simulink model "MTTE_TractionControl"  (R2015a)
settings: Solver=ode45  StartTime=0.0  StopTime=10.0  RelTol=1e-3
libraries: simulink x6
settings Model: Creator=Alexander  LastModifiedBy=Alexander

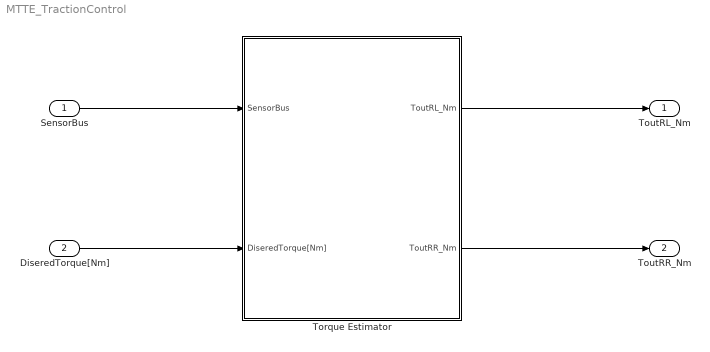
== system MTTE_TractionControl ==
  SensorBus : Inport
  DiseredTorque[Nm] : Inport  Port=2
  Torque Estimator : Subsystem
  ToutRL_Nm : Outport
  ToutRR_Nm : Outport  Port=2
  wires:
  SensorBus/1 -> Torque Estimator/1(SensorBus)
  DiseredTorque[Nm]/1 -> Torque Estimator/2(DiseredTorque[Nm])
  Torque Estimator/1(ToutRL_Nm) -> ToutRL_Nm/1
  Torque Estimator/2(ToutRR_Nm) -> ToutRR_Nm/1

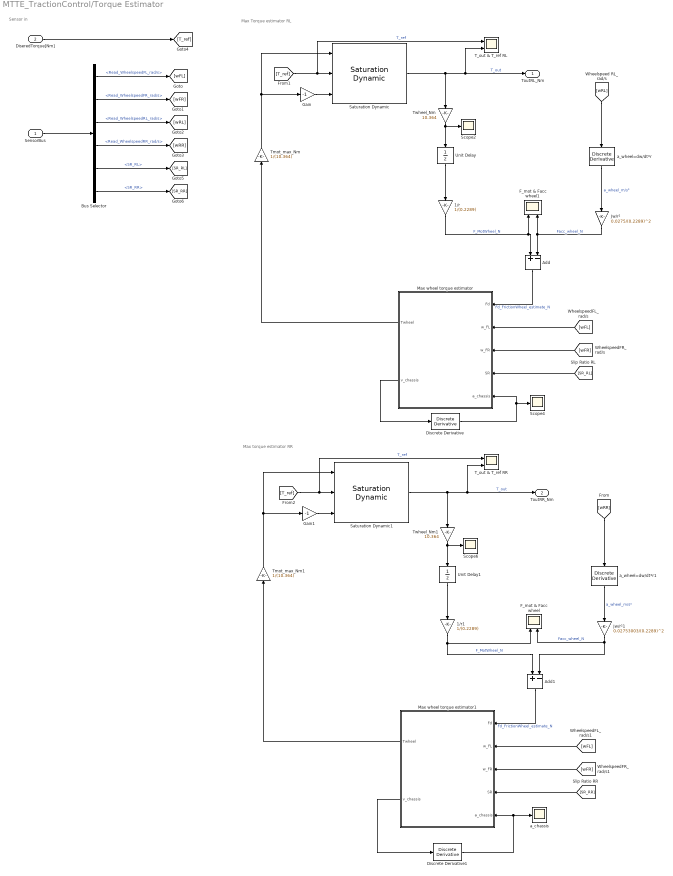
== system MTTE_TractionControl/Torque Estimator ==
  note: Max torque estimator RR
  note: Max Torque estimator RL
  note: Sensor in
  SensorBus : Inport
  DiseredTorque[Nm] : Inport  Port=2
  1/r : Gain  Gain=1/(0.2289)
  1/r1 : Gain  Gain=1/(0.2289)
  Add : Sum  Inputs=+|-
  Add1 : Sum  Inputs=+|-
  Bus Selector : BusSelector  OutputSignals=SensorBus.Read_WheelspeedFL_rad/s,SensorBus.Read_WheelspeedFR_rad/s,SensorBus.Read_WheelspeedRL_rad/s,SensorBus.Read_WheelspeedRR_rad/s,SR_RL,SR_RR
  Discrete Derivative : simulink/Discrete/Discrete Derivative  gainval=1.0  ICPrevScaledInput=0.0  InputProcessing=Inherited  OutMin=[]  OutMax=[]  OutDataType=fixdt(1, 16)  OutScaling=2^-10  DoSatur=off
  Discrete Derivative1 : simulink/Discrete/Discrete Derivative  gainval=1.0  ICPrevScaledInput=0.0  InputProcessing=Inherited  OutMin=[]  OutMax=[]  OutDataType=fixdt(1, 16)  OutScaling=2^-10  DoSatur=off
  F_mot & Facc wheel : Scope  NumInputPorts=2
      settings: YMin=-300~-1755  YMax=600~1755  SaveName=ScopeData23
  F_mot & Facc wheel1 : Scope  NumInputPorts=2
      settings: YMin=250~10  YMax=1750~22  SaveName=ScopeData18
  Gain : Gain  Gain=-1
  Gain1 : Gain  Gain=-1
  Jw/r² : Gain  Gain=0.0275/(0.2289)^2
  Jw/r²1 : Gain  Gain=0.02753003/(0.2289)^2
  Max wheel torque estimator : MATLAB Function  TreatAsAtomicUnit=on
  Max wheel torque estimator1 : MATLAB Function  TreatAsAtomicUnit=on
  Saturation Dynamic : simulink/Discontinuities/Saturation Dynamic  OutMin=[]  OutMax=[]  OutDataTypeStr=Inherit: Same as second input  OutDataType=fixdt(1, 16)  OutScaling=2^-10  DoSatur=off
  Saturation Dynamic1 : simulink/Discontinuities/Saturation Dynamic  OutMin=[]  OutMax=[]  OutDataTypeStr=Inherit: Same as second input  OutDataType=fixdt(1, 16)  OutScaling=2^-10  DoSatur=off
  Scope2 : Scope
      settings: SaveName=ScopeData22
  Scope4 : Scope
      settings: YMin=-10  YMax=10  SaveName=ScopeData24
  Scope6 : Scope
      settings: SaveName=ScopeData26
  T_out & T_ref RL : Scope  NumInputPorts=2
      settings: YMin=-50~-50  YMax=50~50  SaveName=ScopeData17
  T_out & T_ref RR : Scope  NumInputPorts=2
      settings: YMin=-50~-50  YMax=50~50  SaveName=ScopeData28
  Tmot_max_Nm : Gain  Gain=1/(10.364)
  Tmot_max_Nm1 : Gain  Gain=1/(10.364)
  Twheel_Nm : Gain  Gain=10.364
  Twheel_Nm1 : Gain  Gain=10.364
  Unit Delay : UnitDelay  SampleTime=-1
  Unit Delay1 : UnitDelay  SampleTime=-1
  a_chassis : Scope
      settings: YMin=-10  YMax=10  SaveName=ScopeData27
  a_wheel=dw/dt*r : simulink/Discrete/Discrete Derivative  gainval=0.2289  ICPrevScaledInput=0.0  InputProcessing=Inherited  OutMin=[]  OutMax=[]  OutDataType=fixdt(1, 16)  OutScaling=2^-10  DoSatur=off
  a_wheel=dw/dt*r1 : simulink/Discrete/Discrete Derivative  gainval=0.2289  ICPrevScaledInput=0.0  InputProcessing=Inherited  OutMin=[]  OutMax=[]  OutDataType=fixdt(1, 16)  OutScaling=2^-10  DoSatur=off
  ToutRL_Nm : Outport
  ToutRR_Nm : Outport  Port=2
  wires:
  Max wheel torque estimator1/2(v_chassis) -> Discrete Derivative1/1
  [SR_RL] -> Max wheel torque estimator/4(SR)
  Tmot_max_Nm1/1 -> Gain1/1, Saturation Dynamic1/1
  DiseredTorque[Nm]/1 -> [T_ref]
  Bus Selector/6 -> [SR_RR]  "<SR_RR>"
  Gain1/1 -> Saturation Dynamic1/3
  Unit Delay/1 -> 1/r/1
  Bus Selector/4 -> [wRR]  "<Read_WheelspeedRR_rad/s>"
  Bus Selector/5 -> [SR_RL]  "<SR_RL>"
  [wFR] -> Max wheel torque estimator/3(w_FR)
  Twheel_Nm/1 -> Scope2/1, Unit Delay/1
  Unit Delay1/1 -> 1/r1/1
  Gain/1 -> Saturation Dynamic/3
  Max wheel torque estimator1/1(Twheel) -> Tmot_max_Nm1/1
  Saturation Dynamic/1 -> Twheel_Nm/1, ToutRL_Nm/1, T_out & T_ref RL/2  "T_out"
  [SR_RR] -> Max wheel torque estimator1/4(SR)
  Jw/r²1/1 -> Add1/2, F_mot & Facc wheel/2  "Facc_wheel_N"
  Discrete Derivative1/1 -> a_chassis/1, Max wheel torque estimator1/5(a_chassis)
  Bus Selector/3 -> [wRL]  "<Read_WheelspeedRL_rad/s>"
  [wRR] -> a_wheel=dw/dt*r1/1
  Twheel_Nm1/1 -> Scope6/1, Unit Delay1/1
  Add1/1 -> Max wheel torque estimator1/1(Fd)  "Fd_FrictionWheel_estimate_N"
  [T_ref] -> Saturation Dynamic1/2, T_out & T_ref RR/1  "T_ref"
  Saturation Dynamic1/1 -> Twheel_Nm1/1, ToutRR_Nm/1, T_out & T_ref RR/2  "T_out"
  SensorBus/1 -> Bus Selector/1
  Bus Selector/1 -> [wFL]  "<Read_WheelspeedFL_rad/s>"
  Bus Selector/2 -> [wFR]  "<Read_WheelspeedFR_rad/s>"
  [wFL] -> Max wheel torque estimator1/2(w_FL)
  [wFR] -> Max wheel torque estimator1/3(w_FR)
  [T_ref] -> Saturation Dynamic/2, T_out & T_ref RL/1  "T_ref"
  Tmot_max_Nm/1 -> Gain/1, Saturation Dynamic/1
  Max wheel torque estimator/2(v_chassis) -> Discrete Derivative/1
  Discrete Derivative/1 -> Max wheel torque estimator/5(a_chassis), Scope4/1
  Max wheel torque estimator/1(Twheel) -> Tmot_max_Nm/1
  [wRL] -> a_wheel=dw/dt*r/1
  [wFL] -> Max wheel torque estimator/2(w_FL)
  a_wheel=dw/dt*r1/1 -> Jw/r²1/1  "a_wheel_m/s²"
  1/r/1 -> F_mot & Facc wheel1/1, Add/1  "F_MotWheel_N"
  Add/1 -> Max wheel torque estimator/1(Fd)  "Fd_FrictionWheel_estimate_N"
  1/r1/1 -> F_mot & Facc wheel/1, Add1/1  "F_MotWheel_N"
  Jw/r²/1 -> Add/2, F_mot & Facc wheel1/2  "Facc_wheel_N"
  a_wheel=dw/dt*r/1 -> Jw/r²/1  "a_wheel_m/s²"

== matlab function MTTE_TractionControl/Torque Estimator/Max wheel torque estimator1 ==
  data: Fd input; Twheel output; w_FL input; w_FR input; SR input; a_chassis input; v_chassis output
function [Twheel,v_chassis] = TorqueEstimation(Fd,w_FL,w_FR,SR,a_chassis)
%% estimator wheel torque

Jw =0.0275; %[kgm²] Massatraagheid wiel (roterende componenten)
r=0.2286; %[m] straal wiel
a=0.9; %relacation factor a=Vchasis/Vwheel

Tmax= 400; %[Nm] Wheel Torque

w_chassis=(w_FL+w_FR)/2; % average speed
v_chassis=w_chassis*r; %[m/s] velocity of the chasis

if SR <0.08
    Twheel=Tmax;
else
    Twheel = max(a_chassis*Jw/(a*r)+r*Fd,100);
end

== matlab function MTTE_TractionControl/Torque Estimator/Max wheel torque estimator ==
  data: Fd input; Twheel output; w_FL input; w_FR input; SR input; a_chassis input; v_chassis output
function [Twheel,v_chassis] = TorqueEstimation(Fd,w_FL,w_FR,SR,a_chassis)
%% estimator wheel torque

Jw =0.0275; %[kgm²] Massatraagheid wiel (roterende componenten)
r=0.2286; %[m] straal wiel
a=0.9; %relacation factor a=Vchasis/Vwheel

Tmax= 400; %[Nm] Wheel Torque

w_chassis=(w_FL+w_FR)/2; % average speed
v_chassis=w_chassis*r; %[m/s] velocity of the chasis

if SR <0.08
    Twheel=Tmax;
else
    Twheel = max(a_chassis*Jw/(a*r)+r*Fd,100);
end
